simulink model "VCU"  (R2016b)
settings: Solver=ode3  StartTime=0.0  StopTime=1500  RelTol=1e-3
InitFcn:
  | % Call parameters initialization function
  | run optiTruck_init_sim.m;
StopFcn:
  | optiTruck_post_sim;
  | optiTruck_plot_sim;
settings Model: Creator=engin  LastModifiedBy=engin.ozatay
settings DataIOCC: SaveFormat=StructureWithTime  SaveOutput=off  SaveTime=off
settings OptimizationCC: BlockReduction=off  BufferReuse=off  LifeSpan=inf
settings DebuggingCC: AlgebraicLoopMsg=none  UnconnectedInputMsg=none  UnconnectedOutputMsg=none  UnconnectedLineMsg=none  SFExecutionAtInitializationDiag=none
settings HardwareCC: ProdBitPerSizeT=32  ProdBitPerPtrDiffT=32  ProdWordSize=32  ProdHWDeviceType=Specified

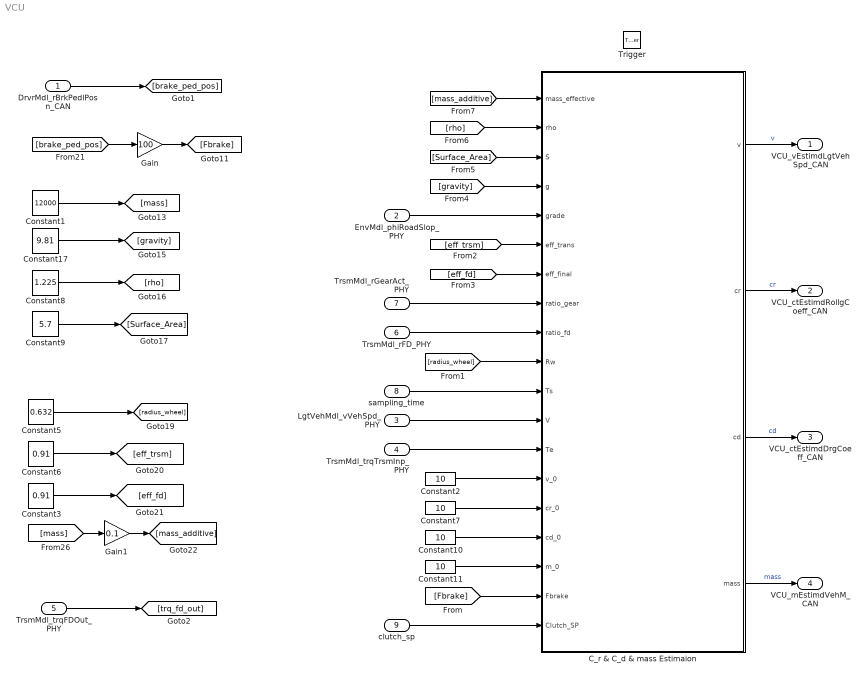
== system VCU ==
  DrvrMdl_rBrkPedlPosn_CAN : Inport
  EnvMdl_phiRoadSlop_PHY : Inport  Port=2
  LgtVehMdl_vVehSpd_PHY : Inport  Port=3
  TrsmMdl_trqTrsmInp_PHY : Inport  Port=4
  TrsmMdl_trqFDOut_PHY : Inport  Port=5
  TrsmMdl_rFD_PHY : Inport  Port=6
  TrsmMdl_rGearAct_PHY : Inport  Port=7
  sampling_time : Inport  Port=8
  clutch_sp : Inport  Port=9
  Trigger : TriggerPort  TriggerType=function-call  VariantControl=Variant  PortDimensions=1
  C_r & C_d & mass Estimaion : MATLAB Function  TreatAsAtomicUnit=on
  Constant1 : Constant  Value=12000
  Constant{2,7,10..11} (4 alike) : Constant  Value=10
  Constant17 : Constant  Value=9.81
  Constant3 : Constant  Value=0.91
  Constant5 : Constant  Value=0.632
  Constant6 : Constant  Value=0.91
  Constant8 : Constant  Value=1.225
  Constant9 : Constant  Value=5.7
  Gain : Gain  Gain=100
  Gain1 : Gain  Gain=0.1
  VCU_vEstimdLgtVehSpd_CAN : Outport
  VCU_ctEstimdRollgCoeff_CAN : Outport  Port=2
  VCU_ctEstimdDrgCoeff_CAN : Outport  Port=3
  VCU_mEstimdVehM_CAN : Outport  Port=4
  wires:
  C_r & C_d & mass Estimaion/3(cd) -> VCU_ctEstimdDrgCoeff_CAN/1  "cd"
  C_r & C_d & mass Estimaion/2(cr) -> VCU_ctEstimdRollgCoeff_CAN/1  "cr"
  TrsmMdl_rGearAct_PHY/1 -> C_r & C_d & mass Estimaion/8(ratio_gear)
  TrsmMdl_rFD_PHY/1 -> C_r & C_d & mass Estimaion/9(ratio_fd)
  EnvMdl_phiRoadSlop_PHY/1 -> C_r & C_d & mass Estimaion/5(grade)
  C_r & C_d & mass Estimaion/1(v) -> VCU_vEstimdLgtVehSpd_CAN/1  "v"
  C_r & C_d & mass Estimaion/4(mass) -> VCU_mEstimdVehM_CAN/1  "mass"
  sampling_time/1 -> C_r & C_d & mass Estimaion/11(Ts)
  LgtVehMdl_vVehSpd_PHY/1 -> C_r & C_d & mass Estimaion/12(V)
  clutch_sp/1 -> C_r & C_d & mass Estimaion/19(Clutch_SP)
  Constant2/1 -> C_r & C_d & mass Estimaion/14(v_0)
  [Fbrake] -> C_r & C_d & mass Estimaion/18(Fbrake)
  TrsmMdl_trqTrsmInp_PHY/1 -> C_r & C_d & mass Estimaion/13(Te)
  Constant1/1 -> [mass]
  Constant17/1 -> [gravity]
  Constant8/1 -> [rho]
  Constant9/1 -> [Surface_Area]
  [brake_ped_pos] -> Gain/1
  Gain/1 -> [Fbrake]
  Constant5/1 -> [radius_wheel]
  Constant6/1 -> [eff_trsm]
  Constant3/1 -> [eff_fd]
  [mass] -> Gain1/1
  Gain1/1 -> [mass_additive]
  Constant7/1 -> C_r & C_d & mass Estimaion/15(cr_0)
  Constant10/1 -> C_r & C_d & mass Estimaion/16(cd_0)
  Constant11/1 -> C_r & C_d & mass Estimaion/17(m_0)
  [radius_wheel] -> C_r & C_d & mass Estimaion/10(Rw)
  [eff_trsm] -> C_r & C_d & mass Estimaion/6(eff_trans)
  [eff_fd] -> C_r & C_d & mass Estimaion/7(eff_final)
  [gravity] -> C_r & C_d & mass Estimaion/4(g)
  [Surface_Area] -> C_r & C_d & mass Estimaion/3(S)
  [rho] -> C_r & C_d & mass Estimaion/2(rho)
  [mass_additive] -> C_r & C_d & mass Estimaion/1(mass_effective)
  DrvrMdl_rBrkPedlPosn_CAN/1 -> [brake_ped_pos]
  TrsmMdl_trqFDOut_PHY/1 -> [trq_fd_out]

== matlab function VCU/C_r & C_d & mass Estimaion ==
  data: v output; mass_effective input size=1; cr output; cd output; rho input; S input; g input; grade input; eff_trans input; eff_final input; ratio_gear input; ratio_fd input; Rw input; Ts input; V input; Te input; v_0 input; cr_0 input; cd_0 input; m_0 input; Fbrake input; Clutch_SP input; mass output
function [v, cr, cd, mass]    = ExtKalman2(mass_effective, rho, S, g, grade, eff_trans, eff_final, ratio_gear, ratio_fd, Rw, Ts, V, Te, v_0, cr_0, cd_0, m_0,Fbrake, Clutch_SP)

% Define storage for the variables that need to persist
% between time periods.
persistent P xhat Q R


if isempty(P)
   % First time through the code so do some initialization
   xhat = [v_0; cr_0; cd_0; 1/m_0];
   P = diag([100,1,10, 0.000001]);
   Q = diag([1^2 0.01^2 0.03^2 0.001^2]);
   R = diag(0.001);
end

if Fbrake >0 || Clutch_SP == 1
    %Q = diag([10^10 0.0001^2 0.0001^2]);
    Q = diag([10^10 0.01^2 0.1^2 0.001^2]);
else
    %Q = diag([1^2 0.0001^2 0.0001^2]);
    Q = diag([1^2 0.01^2 0.1^2 0.001^2]);
end

% Calculate the Jacobians for the state and measurement equations


F = [ 1 - Ts*rho*S*xhat(3)*xhat(1)*xhat(4)/(1 + xhat(4)*mass_effective),   -Ts*g*cos(grade)/(1 + xhat(4)*mass_effective),  -Ts*0.5*rho*S*xhat(4)*xhat(1)*xhat(1)/(1 + xhat(4)*mass_effective), ...
      Ts*(ratio_gear*ratio_fd*eff_trans*eff_final*Te/Rw - 0.5*rho*S*xhat(3)*xhat(1)*xhat(1) + g*sin(grade)*mass_effective + g*cos(grade)*xhat(2)*mass_effective)/(1 + xhat(4)*mass_effective)^2 ;
      0,  1,  0, 0;
      0,  0,  1, 0;
      0,  0,  0, 1];

H = [1 0 0 0];

% Propogate the state and covariance matrices
xhat = [xhat(1) + Ts*(ratio_gear*ratio_fd*eff_trans*eff_final*xhat(4)*Te/Rw - g*sin(grade) - g*cos(grade)*xhat(2) - 0.5*rho*S*xhat(3)*xhat(4)*xhat(1)*xhat(1))/(1 + xhat(4)*mass_effective);
        xhat(2);
        xhat(3);
        xhat(4)];
    
P = F*P*F' + Q;

% Calculate the Kalman gain
K = P*H'/(H*P*H' + R);

% Calculate the measurement residual
z = V; 
resid = z - xhat(1);

% Update the state and covariance estimates
xhat = xhat + K*resid;
P = (eye(size(K,1))-K*H)*P;
% Post the results
v    = xhat(1);
cr   = xhat(2);
cd   = xhat(3);
mass = 1/xhat(4);
